simulink model "CNNCOntrol"  (R2021a)
settings: Solver=VariableStepAuto  StartTime=0.0  StopTime=10.0  RelTol=1e-3
model workspace (MAT data in the model file):
  y0 = 3.14259265359
settings Model: Creator=marti  LastModifiedBy=marti

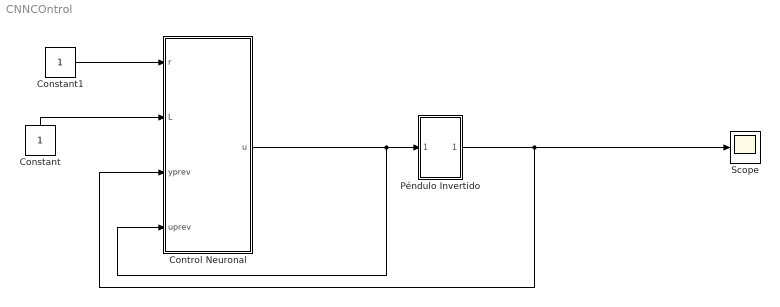
== system CNNCOntrol ==
  Constant : Constant
  Constant1 : Constant
  Control Neuronal : MATLAB Function  TreatAsAtomicUnit=on
  Péndulo Invertido : Subsystem
  Scope : Scope
  wires:
  Constant1/1 -> Control Neuronal/1(r)
  Control Neuronal/1(u) -> Control Neuronal/4(uprev), Péndulo Invertido/1(In1)
  Péndulo Invertido/1(yprev) -> Scope/1, Control Neuronal/3(yprev)
  Constant/1 -> Control Neuronal/2(L)

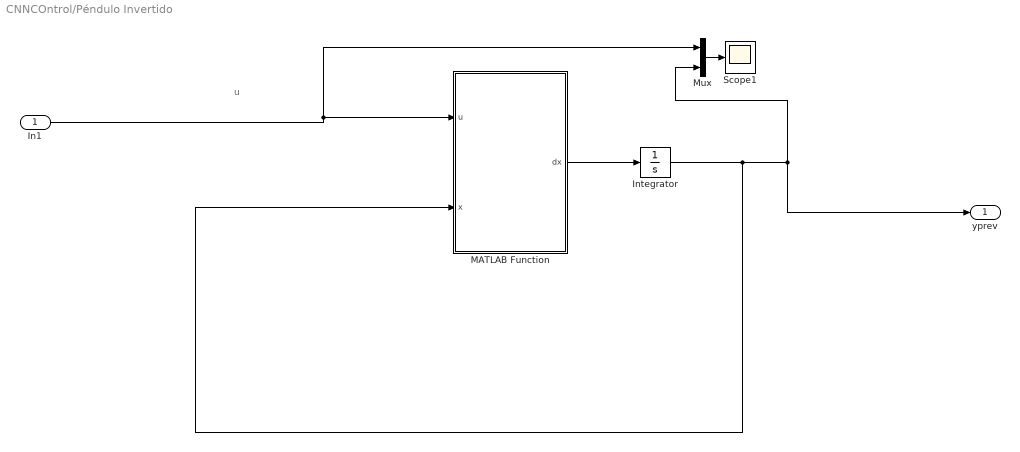
== system CNNCOntrol/Péndulo Invertido ==
  note: u
  In1 : Inport
  Integrator : Integrator  InitialCondition=y0
  MATLAB Function : MATLAB Function  TreatAsAtomicUnit=on
  Mux : Mux  Inputs=2
  Scope1 : Scope
  yprev : Outport
  wires:
  MATLAB Function/1(dx) -> Integrator/1
  In1/1 -> Mux/1, MATLAB Function/1(u)
  Integrator/1 -> MATLAB Function/2(x), yprev/1, Mux/2
  Mux/1 -> Scope1/1

== matlab function CNNCOntrol/Péndulo Invertido/MATLAB Function ==
  data: u input; x input; dx output
function dx = pendcart(u,x)
%x=[x,dx,theta,dtheta]


m = 1;
M = 5;
L = 2;
g = -9.8;
d = 1;


Sx = sin(x(3));
Cx = cos(x(3));
D = L*(M+m*(1-Cx^2));

dx=[x(2);(1/D)*(-m*L*g*Cx*Sx + L*(m*L*x(4)^2*Sx - d*x(2)) + L*u);...
    x(4);(1/D)*((m+M)*g*Sx - Cx*(m*L*x(4)^2*Sx - d*x(2)) - Cx*u)];

== matlab function CNNCOntrol/Control Neuronal ==
  data: r input; u output; L input; yprev input; uprev input
function u = CNN(r, L, yprev, uprev)
y0 = pi + 0.001
u = 1;
end
